simulink model "OpenLoop_Test"  (R2022b)
settings: Solver=VariableStepAuto  StartTime=0.0  StopTime=10.0  RelTol=1e-3
libraries: cstblocks x2
settings Model: Creator=antoninrenoir  LastModifiedBy=antoninrenoir

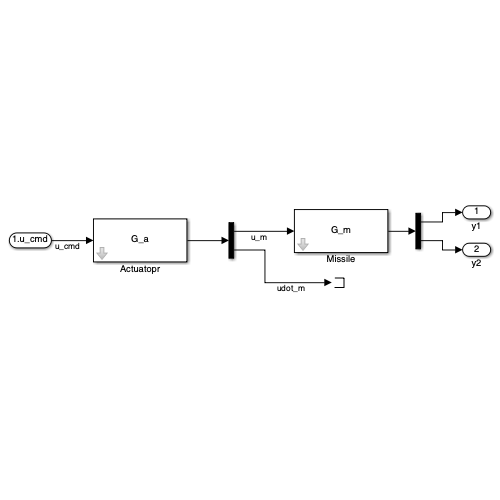
[thumbnail: Simulink's stored preview of the top-level diagram]
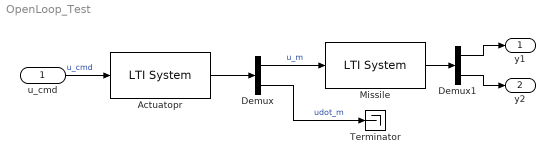
== system OpenLoop_Test ==
  u_cmd : Inport
  Actuatopr : cstblocks/LTI System  sys=G_a  IC=[]
  Demux : Demux  Outputs=2
  Demux1 : Demux  Outputs=2
  Missile : cstblocks/LTI System  sys=G_m  IC=[]
  Terminator : Terminator
  y1 : Outport
  y2 : Outport  Port=2
  wires:
  Demux/1 -> Missile/1  "u_m"
  Missile/1 -> Demux1/1
  Actuatopr/1 -> Demux/1
  Demux/2 -> Terminator/1  "udot_m"
  u_cmd/1 -> Actuatopr/1  "u_cmd"
  Demux1/1 -> y1/1
  Demux1/2 -> y2/1
